simulink model "BUP_FOR_GUI"  (R2018a)
settings: Solver=ode3  StartTime=0.0  StopTime=1000  FixedStep=1  MinStep=1e-8  RelTol=1e-8
undefined symbols (not defined in the file or in its folder): DiscIntNeverNeededParam
libraries: BupSimulinkLibraries x22, simulink_extras x11, SignalEditorBlockLib x2
(part 1 of 2)
settings Model: EnablePacing=on  PacingRate=10  Creator=Юзер33  LastModifiedBy=User33
settings DataIOCC: SaveFormat=Array  OutputSaveName=P_lon
settings OptimizationCC: DefaultParameterBehavior=Inlined  UseDivisionForNetSlopeComputation=on  UseFloatMulNetSlope=on  InlineInvariantSignals=on  PassReuseOutputArgsAs=Individual arguments  ZeroExternalMemoryAtStartup=off  ZeroInternalMemoryAtStartup=off  NoFixptDivByZeroProtection=on  EfficientFloat2IntCast=on  LifeSpan=1  OptimizationLevel=level1  OptimizationCustomize=off
settings DebuggingCC: ParameterTunabilityLossMsg=error
settings HardwareCC: ProdBitPerPointer=32  ProdBitPerSizeT=32  ProdBitPerPtrDiffT=32  ProdLargestAtomicInteger=Long  ProdLargestAtomicFloat=Double  ProdWordSize=32  ProdLongLongMode=on  ProdHWDeviceType=ARM Compatible->ARM Cortex
settings SFSimCC: MATLABDynamicMemAlloc=off
settings RTWCC: SystemTargetFile=ert.tlc  GenCodeOnly=on  PackageGeneratedCodeAndArtifacts=on  PackageName=BupModel  TemplateMakefile=ert_default_tmf  GenerateReport=on  RTWVerbose=off  BuildConfiguration=Faster Runs  IncludeHyperlinkInReport=on  LaunchReport=on  GenerateTraceInfo=on  GenerateTraceReport=on  GenerateTraceReportSl=on  GenerateTraceReportSf=on  GenerateTraceReportEml=on  GenerateWebview=on  GenerateCodeMetricsReport=on  GenerateCodeReplacementReport=on
settings CodeAppCC: ForceParamTrailComments=on  IgnoreCustomStorageClasses=off  OperatorAnnotations=on  SimulinkDataObjDesc=on  SFDataObjDesc=on  MATLABFcnDesc=on  CustomSymbolStrGlobalVar=Easy_reg_$N$M  CustomSymbolStrType=$N$M  CustomSymbolStrFcn=$N$M$F  CustomSymbolStrMacro=$N$M  InsertBlockDesc=on  StateflowObjectComments=on  MATLABSourceComments=on  ReqsInCode=on
settings ERTTargetCC: TargetLangStandard=C99 (ISO)  GenerateSampleERTMain=on  IncludeMdlTerminateFcn=off  CombineSignalStateStructs=on  SupportComplex=off  SupportNonInlinedSFcns=on  InlinedParameterPlacement=NonHierarchical  RootIOFormat=Structure reference  ERTCustomFileTemplate=example_file_process.tlc  ERTFilePackagingFormat=CompactWithDataFile

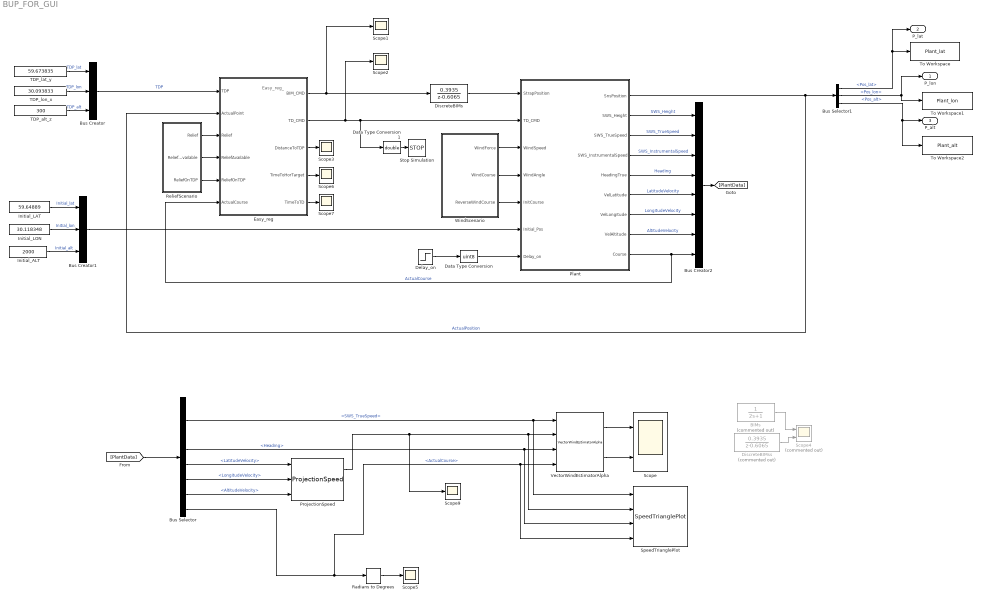
== system BUP_FOR_GUI ==
  note: Easy_reg_
  BIMs : TransferFcn  Commented=on  Denominator=[2 1]
  Bus Creator : BusCreator  Inputs=3
  Bus Creator1 : BusCreator  Inputs=3
  Bus Creator2 : BusCreator  Inputs=8
  Bus Selector : BusSelector  OutputSignals=SWS_Height,SWS_TrueSpeed,SWS_InstrumentalSpeed,Heading,LatitudeVelocity,LongitudeVelocity,AltitudeVelocity,ActualCourse
  Bus Selector1 : BusSelector  OutputSignals=Pos_lat,Pos_lon,Pos_alt
  Data Type Conversion : DataTypeConversion  OutDataTypeStr=uint8
  Data Type Conversion1 : DataTypeConversion  OutDataTypeStr=double
  Delay_on : Step  Time=20  SampleTime=0
  DiscreteBIMs : DiscreteTransferFcn  Numerator=[0.3935]  Denominator=[1 -0.6065]
  DiscreteBIMss : DiscreteTransferFcn  Commented=on  Numerator=[0.3935]  Denominator=[1 -0.6065]
  Easy_reg : Subsystem  TreatAsAtomicUnit=on  SystemSampleTime=1
  Initial_ALT : Constant  Value=2000
  Initial_LAT : Constant  Value=59.64889
  Initial_LON : Constant  Value=30.118348
  Plant : Subsystem  TreatAsAtomicUnit=on
  ProjectionSpeed : BupSimulinkLibraries/ProjectionSpeed
  Radians to Degrees : simulink_extras/Transformations/Radians to Degrees
  ReliefScenario : Subsystem  SystemSampleTime=1
  Scope : Scope  NumInputPorts=2
  Scope{1..3,5..7,9} (7 alike) : Scope
  Scope4 : Scope  Commented=on  NumInputPorts=2
  SpeedTrianglePlot : BupSimulinkLibraries/SpeedTrianglePlot
  Stop Simulation : Stop
  TDP_alt_z : Constant  Value=300
  TDP_lat_y : Constant  Value=59.673835
  TDP_lon_x : Constant  Value=30.093833
  To Workspace : ToWorkspace  VariableName=Plant_lat  SampleTime=-1
  To Workspace1 : ToWorkspace  VariableName=Plant_lon  SampleTime=-1
  To Workspace2 : ToWorkspace  VariableName=Plant_alt  SampleTime=-1
  VectorWindEstimatorAlpha : BupSimulinkLibraries/VectorWindEstimatorAlpha  SystemSampleTime=-1
  WindScenario : Subsystem  SystemSampleTime=1
  P_lon : Outport
  P_lat : Outport  Port=2
  P_alt : Outport  Port=3
  wires:
  TDP_alt_z/1 -> Bus Creator/3  "TDP_alt"
  TDP_lon_x/1 -> Bus Creator/2  "TDP_lon"
  TDP_lat_y/1 -> Bus Creator/1  "TDP_lat"
  Bus Creator/1 -> Easy_reg/1(TDP)  "TDP"
  Plant/1(SnsPosition) -> Easy_reg/2(ActualPoint), Bus Selector1/1  "ActualPosition"
  Initial_LAT/1 -> Bus Creator1/1  "Initial_lat"
  Bus Creator1/1 -> Plant/6(Initial_Pos)
  Initial_LON/1 -> Bus Creator1/2  "Initial_lon"
  Initial_ALT/1 -> Bus Creator1/3  "Initial_alt"
  BIMs/1 -> Scope4/1
  DiscreteBIMss/1 -> Scope4/2
  Bus Selector1/1 -> To Workspace/1, P_lat/1  "<Pos_lat>"
  Delay_on/1 -> Data Type Conversion/1
  ReliefScenario/3(ReliefOnTDP) -> Easy_reg/5(ReliefOnTDP)
  ReliefScenario/1(Relief) -> Easy_reg/3(Relief)
  ReliefScenario/2(ReliefAvailable) -> Easy_reg/4(ReliefAvailable)
  DiscreteBIMs/1 -> Plant/1(StrapPosition)
  Easy_reg/1(BIM_CMD) -> DiscreteBIMs/1, Scope1/1
  Easy_reg/2(TD_CMD) -> Scope2/1, Data Type Conversion1/1, Plant/2(TD_CMD)
  Data Type Conversion/1 -> Plant/7(Delay_on)
  Bus Selector1/2 -> P_lon/1, To Workspace1/1  "<Pos_lon>"
  Bus Selector1/3 -> To Workspace2/1, P_alt/1  "<Pos_alt>"
  Plant/7(VelLongitude) -> Bus Creator2/6  "LongitudeVelocity"
  Plant/8(VelAltitude) -> Bus Creator2/7  "AltitudeVelocity"
  Plant/6(VelLatitude) -> Bus Creator2/5  "LatitudeVelocity"
  Plant/2(SWS_Height) -> Bus Creator2/1  "SWS_Height"
  Plant/5(HeadingTrue) -> Bus Creator2/4  "Heading"
  Plant/4(SWS_InstrumentalSpeed) -> Bus Creator2/3  "SWS_InstrumentalSpeed"
  Bus Creator2/1 -> [PlantData]
  Plant/9(Course) -> Easy_reg/6(ActualCourse), Bus Creator2/8  "ActualCourse"
  Plant/3(SWS_TrueSpeed) -> Bus Creator2/2  "SWS_TrueSpeed"
  WindScenario/2(WindCourse) -> Plant/4(WindAngle)
  WindScenario/1(WindForce) -> Plant/3(WindSpeed)
  WindScenario/3(ReverseWindCourse) -> Plant/5(InitCourse)
  [PlantData] -> Bus Selector/1
  Bus Selector/6 -> ProjectionSpeed/2  "<LongitudeVelocity>"
  Bus Selector/2 -> SpeedTrianglePlot/1, VectorWindEstimatorAlpha/1  "<SWS_TrueSpeed>"
  Radians to Degrees/1 -> Scope5/1
  Bus Selector/8 -> SpeedTrianglePlot/4, VectorWindEstimatorAlpha/4, Radians to Degrees/1  "<ActualCourse>"
  Bus Selector/4 -> SpeedTrianglePlot/3, VectorWindEstimatorAlpha/3  "<Heading>"
  VectorWindEstimatorAlpha/1 -> Scope/1
  VectorWindEstimatorAlpha/2 -> Scope/2
  ProjectionSpeed/1 -> Scope9/1, SpeedTrianglePlot/2, VectorWindEstimatorAlpha/2
  Bus Selector/5 -> ProjectionSpeed/1  "<LatitudeVelocity>"
  Bus Selector/7 -> ProjectionSpeed/3  "<AltitudeVelocity>"
  Data Type Conversion1/1 -> Stop Simulation/1
  Easy_reg/3(DistanceToTDP) -> Scope3/1
  Easy_reg/4(TimeToHorTarget) -> Scope6/1
  Easy_reg/5(TimeToTD) -> Scope7/1

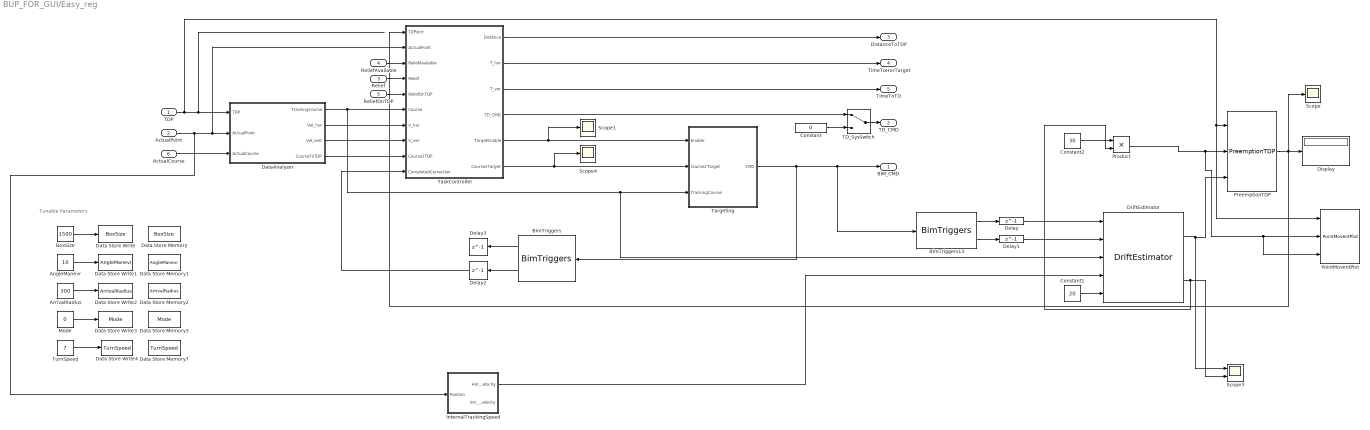
== system BUP_FOR_GUI/Easy_reg ==
  note: Tunable Parameters
  TDP : Inport
  ActualPoint : Inport  Port=2
  Relief : Inport  Port=3
  ReliefAvailable : Inport  Port=4
  ReliefOnTDP : Inport  Port=5
  ActualCourse : Inport  Port=6
  AngleManevr : Constant  Value=10
  ArrivalRadius : Constant  Value=300
  BimTriggers : BupSimulinkLibraries/BimTriggers
  BimTriggers13 : BupSimulinkLibraries/BimTriggers
  BoxSize : Constant  Value=1500
  Constant : Constant  Value=0
  Constant1 : Constant  Value=20
  Constant2 : Constant  Value=30
  Data Store Memory : DataStoreMemory  DataStoreName=BoxSize  ReadBeforeWriteMsg=warning  WriteAfterWriteMsg=warning  WriteAfterReadMsg=warning  ShowAdditionalParam=off  OutDataTypeStr=double  Dimensions=1
  Data Store Memory1 : DataStoreMemory  DataStoreName=AngleManevr  ReadBeforeWriteMsg=warning  WriteAfterWriteMsg=warning  WriteAfterReadMsg=warning  ShowAdditionalParam=off  OutDataTypeStr=double  Dimensions=1
  Data Store Memory2 : DataStoreMemory  DataStoreName=ArrivalRadius  ReadBeforeWriteMsg=warning  WriteAfterWriteMsg=warning  WriteAfterReadMsg=warning  ShowAdditionalParam=off  OutDataTypeStr=double  Dimensions=1
  Data Store Memory3 : DataStoreMemory  DataStoreName=Mode  ReadBeforeWriteMsg=warning  WriteAfterWriteMsg=warning  WriteAfterReadMsg=warning  ShowAdditionalParam=off  OutDataTypeStr=uint8  Dimensions=1
  Data Store Memory7 : DataStoreMemory  DataStoreName=TurnSpeed  ReadBeforeWriteMsg=warning  WriteAfterWriteMsg=warning  WriteAfterReadMsg=warning  ShowAdditionalParam=off  OutDataTypeStr=double  Dimensions=1
  Data Store Write : DataStoreWrite  DataStoreName=BoxSize
  Data Store Write1 : DataStoreWrite  DataStoreName=AngleManevr
  Data Store Write2 : DataStoreWrite  DataStoreName=ArrivalRadius
  Data Store Write3 : DataStoreWrite  DataStoreName=Mode
  Data Store Write4 : DataStoreWrite  DataStoreName=TurnSpeed
  DataAnalyzer : Subsystem
  Delay : Delay  DelayLength=1
  Delay1 : Delay  DelayLength=1
  Delay2 : Delay  DelayLength=1  InitialCondition=0
  Delay3 : Delay  DelayLength=1  InitialCondition=0
  Display : Display
  DriftEstimator : BupSimulinkLibraries/DriftEstimator
  InternalTrackingSpeed : Subsystem
  Mode : Constant  Value=0  OutDataTypeStr=uint8
  PointMoventPlot : BupSimulinkLibraries/PointMoventPlot
  PreemptionTDP : BupSimulinkLibraries/PreemptionTDP
  Product : Product
  Scope : Scope
  Scope1 : Scope
  Scope3 : Scope  NumInputPorts=2
  Scope4 : Scope
  TD_SysSwitch : ManualSwitch
  Targeting : Subsystem
  TaskController : Stateflow chart  TreatAsAtomicUnit=on  SystemSampleTime=1
  TurnSpeed : Constant  Value=7  OutDataTypeStr=double
  BIM_CMD : Outport
  TD_CMD : Outport  Port=2  OutDataTypeStr=uint8
  DistanceToTDP : Outport  Port=3
  TimeToHorTarget : Outport  Port=4
  TimeToTD : Outport  Port=5
  wires:
  TaskController/4(TD_CMD) -> TD_SysSwitch/1
  BoxSize/1 -> Data Store Write/1
  AngleManevr/1 -> Data Store Write1/1
  ArrivalRadius/1 -> Data Store Write2/1
  TD_SysSwitch/1 -> TD_CMD/1
  Constant/1 -> TD_SysSwitch/2
  Mode/1 -> Data Store Write3/1
  TurnSpeed/1 -> Data Store Write4/1
  TaskController/5(TargetEnable) -> Scope1/1, Targeting/1(Enable)
  DataAnalyzer/2(Vel_hor) -> TaskController/7(V_hor)
  DataAnalyzer/3(Vel_vert) -> TaskController/8(V_ver)
  ActualCourse/1 -> DataAnalyzer/3(ActualCourse)
  ReliefAvailable/1 -> TaskController/3(ReliefAvailable)
  Relief/1 -> TaskController/4(Relief)
  ReliefOnTDP/1 -> TaskController/5(ReliefOnTDP)
  TaskController/1(Distance) -> DistanceToTDP/1
  TaskController/2(T_hor) -> TimeToHorTarget/1
  TaskController/3(T_ver) -> TimeToTD/1
  ActualPoint/1 -> InternalTrackingSpeed/1(Position), DataAnalyzer/2(ActualPoint), TaskController/2(ActualPoint)
  TaskController/6(Course2Target) -> Scope4/1, Targeting/2(Course2Target)
  Targeting/1(CMD) -> BimTriggers/1, BimTriggers13/1, BIM_CMD/1
  Delay/1 -> DriftEstimator/1
  Delay1/1 -> DriftEstimator/2
  DriftEstimator/2 -> Product/2, Scope3/2
  BimTriggers13/2 -> Delay1/1
  BimTriggers13/1 -> Delay/1
  BimTriggers/2 -> Delay2/1
  TDP/1 -> PointMoventPlot/1, PreemptionTDP/1, DataAnalyzer/1(TDP)
  DataAnalyzer/1(TrackingCourse) -> DriftEstimator/3, Targeting/3(TrackingCourse), TaskController/6(Course)
  InternalTrackingSpeed/1(Hor_Velocity) -> DriftEstimator/4
  DataAnalyzer/4(CourseToTDP) -> TaskController/9(Course2TDP)
  DriftEstimator/1 -> PreemptionTDP/3, Scope3/1
  Constant1/1 -> DriftEstimator/5
  BimTriggers/1 -> Delay3/1
  Delay2/1 -> TaskController/10(CompletedCorrection)
  Constant2/1 -> Product/1
  Product/1 -> PointMoventPlot/3, PointMoventPlot/2, PreemptionTDP/2
  PreemptionTDP/1 -> Scope/1, TaskController/1(TDPoint), Display/1

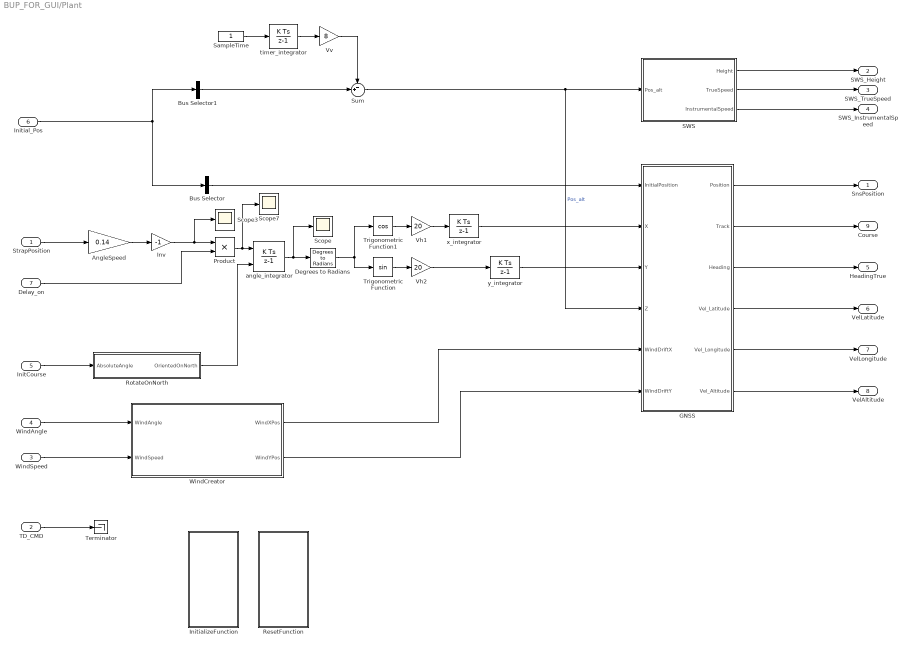
== system BUP_FOR_GUI/Plant ==
  StrapPosition : Inport  OutDataTypeStr=double  PortDimensions=1
  TD_CMD : Inport  Port=2  OutDataTypeStr=uint8  PortDimensions=1
  WindSpeed : Inport  Port=3
  WindAngle : Inport  Port=4
  InitCourse : Inport  Port=5
  Initial_Pos : Inport  Port=6
  Delay_on : Inport  Port=7
  AngleSpeed : Gain  Gain=0.14
  Bus Selector : BusSelector  OutputSignals=Initial_lat,Initial_lon  OutputAsBus=on
  Bus Selector1 : BusSelector  OutputSignals=Initial_alt  OutputAsBus=on
  Degrees to Radians : simulink_extras/Transformations/Degrees to Radians
  GNSS : Subsystem
  InitializeFunction : Subsystem  TreatAsAtomicUnit=on
  Inv : Gain  Gain=-1
  Product : Product
  ResetFunction : Subsystem  TreatAsAtomicUnit=on
  RotateOnNorth : Subsystem
  SWS : Subsystem
  SampleTime : Constant
  Scope : Scope
  Scope3 : Scope
  Scope7 : Scope
  Sum : Sum  Inputs=-+|
  Terminator : Terminator
  Trigonometric Function : Trigonometry
  Trigonometric Function1 : Trigonometry  Operator=cos
  Vh1 : Gain  Gain=20
  Vh2 : Gain  Gain=20
  Vv : Gain  Gain=8
  WindCreator : Subsystem
  angle_integrator : DiscreteIntegrator  InitialConditionSource=external  InitialCondition=90  SampleTime=-1  ICPrevOutput=DiscIntNeverNeededParam  ICPrevScaledInput=DiscIntNeverNeededParam
  timer_integrator : DiscreteIntegrator  SampleTime=-1  ICPrevOutput=DiscIntNeverNeededParam  ICPrevScaledInput=DiscIntNeverNeededParam
  x_integrator : DiscreteIntegrator  SampleTime=-1  ICPrevOutput=DiscIntNeverNeededParam  ICPrevScaledInput=DiscIntNeverNeededParam
  y_integrator : DiscreteIntegrator  SampleTime=-1  ICPrevOutput=DiscIntNeverNeededParam  ICPrevScaledInput=DiscIntNeverNeededParam
  SnsPosition : Outport
  SWS_Height : Outport  Port=2
  SWS_TrueSpeed : Outport  Port=3
  SWS_InstrumentalSpeed : Outport  Port=4
  HeadingTrue : Outport  Port=5
  VelLatitude : Outport  Port=6
  VelLongitude : Outport  Port=7
  VelAltitude : Outport  Port=8
  Course : Outport  Port=9
  wires:
  Degrees to Radians/1 -> Trigonometric Function1/1, Trigonometric Function/1
  angle_integrator/1 -> Scope/1, Degrees to Radians/1
  Trigonometric Function1/1 -> Vh1/1
  Trigonometric Function/1 -> Vh2/1
  Inv/1 -> Product/1, Scope3/1
  Delay_on/1 -> Product/2
  timer_integrator/1 -> Vv/1
  Vv/1 -> Sum/1
  Sum/1 -> GNSS/4(Z), SWS/1(Pos_alt)  "Pos_alt"
  Initial_Pos/1 -> Bus Selector1/1, Bus Selector/1
  Bus Selector/1 -> GNSS/1(InitialPosition)
  Bus Selector1/1 -> Sum/2
  Vh1/1 -> x_integrator/1
  Vh2/1 -> y_integrator/1
  StrapPosition/1 -> AngleSpeed/1
  Product/1 -> Scope7/1, angle_integrator/1
  AngleSpeed/1 -> Inv/1
  SWS/1(Height) -> SWS_Height/1
  SWS/2(TrueSpeed) -> SWS_TrueSpeed/1
  SWS/3(InstrumentalSpeed) -> SWS_InstrumentalSpeed/1
  SampleTime/1 -> timer_integrator/1
  InitCourse/1 -> RotateOnNorth/1(AbsoluteAngle)
  TD_CMD/1 -> Terminator/1
  WindAngle/1 -> WindCreator/1(WindAngle)
  WindSpeed/1 -> WindCreator/2(WindSpeed)
  RotateOnNorth/1(OrientedOnNorth) -> angle_integrator/2
  x_integrator/1 -> GNSS/2(X)
  y_integrator/1 -> GNSS/3(Y)
  WindCreator/1(WindXPos) -> GNSS/5(WindDriftX)
  WindCreator/2(WindYPos) -> GNSS/6(WindDriftY)
  GNSS/1(Position) -> SnsPosition/1
  GNSS/3(Heading) -> HeadingTrue/1
  GNSS/2(Track) -> Course/1
  GNSS/4(Vel_Latitude) -> VelLatitude/1
  GNSS/5(Vel_Longitude) -> VelLongitude/1
  GNSS/6(Vel_Altitude) -> VelAltitude/1

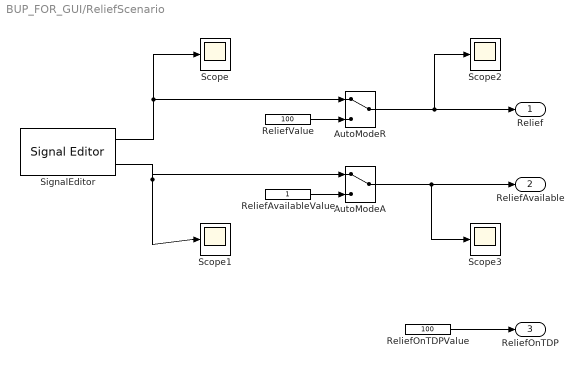
== system BUP_FOR_GUI/ReliefScenario ==
  AutoModeA : ManualSwitch
  AutoModeR : ManualSwitch
  ReliefAvailableValue : Constant  OutDataTypeStr=uint8
  ReliefOnTDPValue : Constant  Value=100  OutDataTypeStr=int16
  ReliefValue : Constant  Value=100  OutDataTypeStr=int16
  Scope{,1..3} (4 alike) : Scope
  SignalEditor : SignalEditorBlockLib/Signal Editor  FileName=ReliefScenario.mat  ActiveScenario=Scenario  ActiveSignal=Relief  IsBus=off  OutputBusObjectStr=Bus: BusObject  SampleTime=-1  ZeroCross=off  OutputAfterFinalValue=Setting to zero  Unit=inherit
  Relief : Outport
  ReliefAvailable : Outport  Port=2
  ReliefOnTDP : Outport  Port=3
  wires:
  SignalEditor/2 -> Scope1/1, AutoModeA/1
  SignalEditor/1 -> Scope/1, AutoModeR/1
  ReliefAvailableValue/1 -> AutoModeA/2
  ReliefValue/1 -> AutoModeR/2
  AutoModeR/1 -> Scope2/1, Relief/1
  AutoModeA/1 -> Scope3/1, ReliefAvailable/1
  ReliefOnTDPValue/1 -> ReliefOnTDP/1

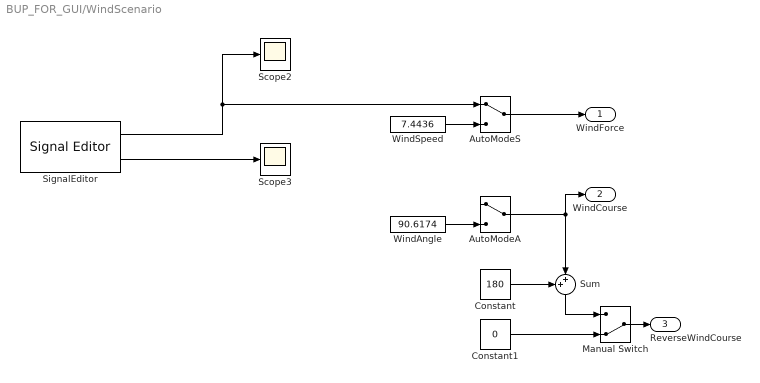
== system BUP_FOR_GUI/WindScenario ==
  AutoModeA : ManualSwitch
  AutoModeS : ManualSwitch
  Constant : Constant  Value=180
  Constant1 : Constant  Value=0
  Manual Switch : ManualSwitch  CurrentSetting=0
  Scope2 : Scope
  Scope3 : Scope
  SignalEditor : SignalEditorBlockLib/Signal Editor  FileName=autoWind.mat  ActiveScenario=Scenario  ActiveSignal=WindSpeed  IsBus=off  OutputBusObjectStr=Bus: BusObject  SampleTime=-1  ZeroCross=off  OutputAfterFinalValue=Setting to zero  Unit=inherit
  Sum : Sum  Inputs=++|
  WindAngle : Constant  Value=90.6174
  WindSpeed : Constant  Value=7.4436
  WindForce : Outport
  WindCourse : Outport  Port=2
  ReverseWindCourse : Outport  Port=3
  wires:
  SignalEditor/1 -> AutoModeS/1, Scope2/1
  WindAngle/1 -> AutoModeA/2
  WindSpeed/1 -> AutoModeS/2
  AutoModeS/1 -> WindForce/1
  AutoModeA/1 -> WindCourse/1, Sum/2
  Sum/1 -> Manual Switch/1
  Constant/1 -> Sum/1
  Manual Switch/1 -> ReverseWindCourse/1
  Constant1/1 -> Manual Switch/2
  SignalEditor/2 -> Scope3/1

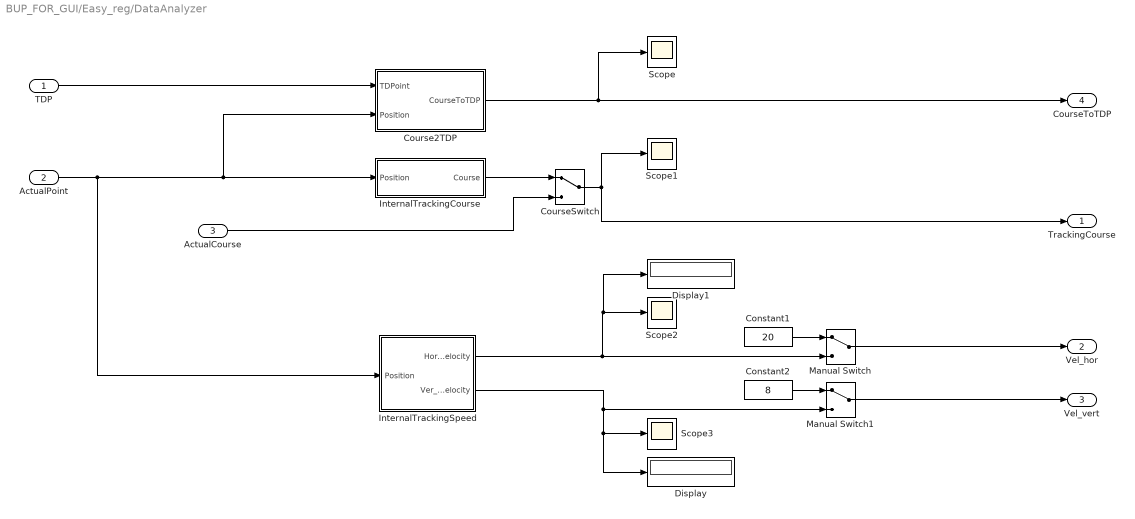
== system BUP_FOR_GUI/Easy_reg/DataAnalyzer ==
  TDP : Inport
  ActualPoint : Inport  Port=2
  ActualCourse : Inport  Port=3
  Constant1 : Constant  Value=20
  Constant2 : Constant  Value=8
  Course2TDP : Subsystem
  CourseSwitch : ManualSwitch
  Display : Display
  Display1 : Display
  InternalTrackingCourse : Subsystem
  InternalTrackingSpeed : Subsystem
  Manual Switch : ManualSwitch
  Manual Switch1 : ManualSwitch
  Scope{,1..3} (4 alike) : Scope
  TrackingCourse : Outport
  Vel_hor : Outport  Port=2
  Vel_vert : Outport  Port=3
  CourseToTDP : Outport  Port=4
  wires:
  CourseSwitch/1 -> TrackingCourse/1, Scope1/1
  TDP/1 -> Course2TDP/1(TDPoint)
  InternalTrackingCourse/1(Course) -> CourseSwitch/1
  ActualCourse/1 -> CourseSwitch/2
  ActualPoint/1 -> InternalTrackingSpeed/1(Position), Course2TDP/2(Position), InternalTrackingCourse/1(Position)
  InternalTrackingSpeed/1(Hor_Velocity) -> Manual Switch/2, Display1/1, Scope2/1
  InternalTrackingSpeed/2(Ver_Velocity) -> Manual Switch1/2, Scope3/1, Display/1
  Manual Switch/1 -> Vel_hor/1
  Constant1/1 -> Manual Switch/1
  Manual Switch1/1 -> Vel_vert/1
  Course2TDP/1(CourseToTDP) -> Scope/1, CourseToTDP/1
  Constant2/1 -> Manual Switch1/1

== system BUP_FOR_GUI/Easy_reg/InternalTrackingSpeed ==
  Position : Inport
  Constant : Constant
  GPSVelocity : BupSimulinkLibraries/GPSVelocity
  LastPos1 : Delay  DelayLength=1
  ProjectionSpeed : BupSimulinkLibraries/ProjectionSpeed
  Hor_Velocity : Outport
  Ver_Velocity : Outport  Port=2
  wires:
  LastPos1/1 -> GPSVelocity/2
  ProjectionSpeed/2 -> Ver_Velocity/1
  Position/1 -> LastPos1/1, GPSVelocity/1
  ProjectionSpeed/1 -> Hor_Velocity/1
  GPSVelocity/1 -> ProjectionSpeed/1
  GPSVelocity/2 -> ProjectionSpeed/2
  GPSVelocity/3 -> ProjectionSpeed/3
  Constant/1 -> GPSVelocity/3

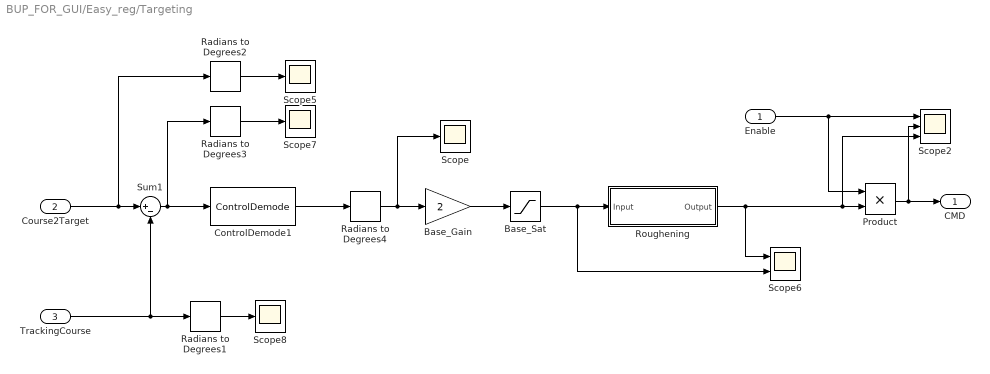
== system BUP_FOR_GUI/Easy_reg/Targeting ==
  Enable : Inport  OutDataTypeStr=uint8  PortDimensions=1
  Course2Target : Inport  Port=2  OutDataTypeStr=double  PortDimensions=1
  TrackingCourse : Inport  Port=3  OutDataTypeStr=double  PortDimensions=1
  Base_Gain : Gain  Gain=2
  Base_Sat : Saturate  UpperLimit=50  LowerLimit=-50
  ControlDemode1 : BupSimulinkLibraries/ControlDemode
  Product : Product
  Radians to Degrees{1..4} (4 alike) : simulink_extras/Transformations/Radians to Degrees
  Roughening : Subsystem
  Scope{,5,7..8} (4 alike) : Scope
  Scope2 : Scope  NumInputPorts=3
  Scope6 : Scope  NumInputPorts=2
  Sum1 : Sum  Inputs=|+-
  CMD : Outport  OutDataTypeStr=double
  wires:
  Course2Target/1 -> Radians to Degrees2/1, Sum1/1
  Radians to Degrees3/1 -> Scope7/1
  Radians to Degrees2/1 -> Scope5/1
  Base_Sat/1 -> Scope6/2, Roughening/1(Input)
  Base_Gain/1 -> Base_Sat/1
  Radians to Degrees4/1 -> Scope/1, Base_Gain/1
  Enable/1 -> Product/1, Scope2/1
  Product/1 -> Scope2/2, CMD/1
  TrackingCourse/1 -> Radians to Degrees1/1, Sum1/2
  Sum1/1 -> ControlDemode1/1, Radians to Degrees3/1
  ControlDemode1/1 -> Radians to Degrees4/1
  Roughening/1(Output) -> Product/2, Scope2/3, Scope6/1
  Radians to Degrees1/1 -> Scope8/1

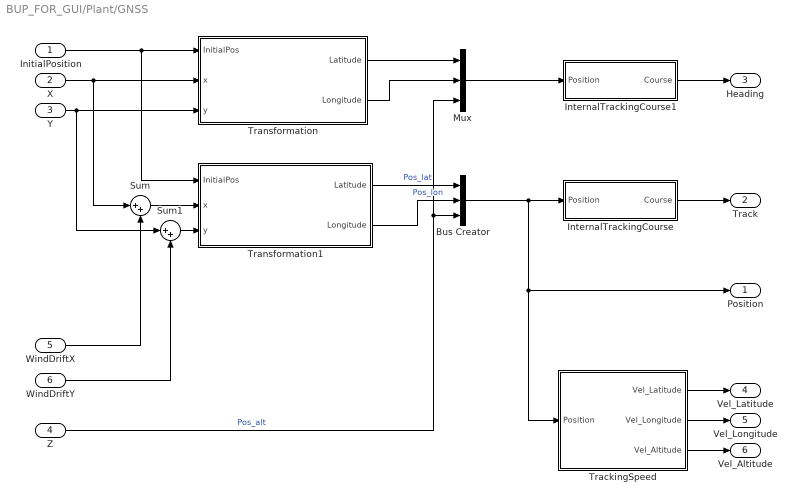
== system BUP_FOR_GUI/Plant/GNSS ==
  InitialPosition : Inport
  X : Inport  Port=2
  Y : Inport  Port=3
  Z : Inport  Port=4
  WindDriftX : Inport  Port=5
  WindDriftY : Inport  Port=6
  Bus Creator : BusCreator  Inputs=3
  InternalTrackingCourse : Subsystem
  InternalTrackingCourse1 : Subsystem
  Mux : Mux  Inputs=3
  Sum : Sum  Inputs=|++
  Sum1 : Sum  Inputs=|++
  TrackingSpeed : Subsystem
  Transformation : Subsystem
  Transformation1 : Subsystem
  Position : Outport
  Track : Outport  Port=2
  Heading : Outport  Port=3
  Vel_Latitude : Outport  Port=4
  Vel_Longitude : Outport  Port=5
  Vel_Altitude : Outport  Port=6
  wires:
  InitialPosition/1 -> Transformation1/1(InitialPos), Transformation/1(InitialPos)
  X/1 -> Sum/1, Transformation/2(x)
  Y/1 -> Sum1/1, Transformation/3(y)
  Sum/1 -> Transformation1/2(x)
  Sum1/1 -> Transformation1/3(y)
  WindDriftX/1 -> Sum/2
  WindDriftY/1 -> Sum1/2
  TrackingSpeed/2(Vel_Longitude) -> Vel_Longitude/1
  TrackingSpeed/3(Vel_Altitude) -> Vel_Altitude/1
  TrackingSpeed/1(Vel_Latitude) -> Vel_Latitude/1
  Transformation/1(Latitude) -> Mux/1
  Transformation/2(Longitude) -> Mux/2
  Mux/1 -> InternalTrackingCourse1/1(Position)
  Transformation1/1(Latitude) -> Bus Creator/1  "Pos_lat"
  Bus Creator/1 -> InternalTrackingCourse/1(Position), TrackingSpeed/1(Position), Position/1
  Z/1 -> Mux/3, Bus Creator/3  "Pos_alt"
  InternalTrackingCourse1/1(Course) -> Heading/1
  InternalTrackingCourse/1(Course) -> Track/1
  Transformation1/2(Longitude) -> Bus Creator/2  "Pos_lon"

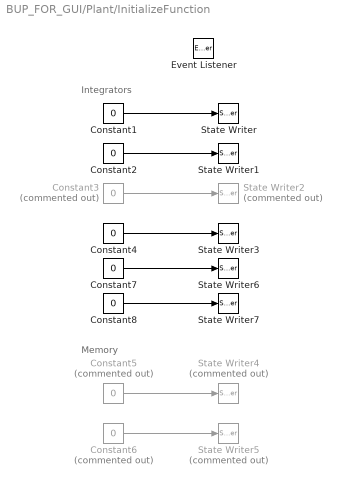
== system BUP_FOR_GUI/Plant/InitializeFunction ==
  note: Memory
  note: Integrators
  Constant{1..2,4,7..8} (5 alike) : Constant  Value=0
  Constant3 : Constant  Commented=on  Value=0
  Constant5 : Constant  Commented=on  Value=0
  Constant6 : Constant  Commented=on  Value=0
  Event Listener : EventListener  DisableCoverage=on  EventName=reset
  State Writer : StateWriter  StateOwnerBlock=../../x_integrator
  State Writer1 : StateWriter  StateOwnerBlock=../../y_integrator
  State Writer2 : StateWriter  Commented=on  StateOwnerBlock=../../angle_integrator
  State Writer3 : StateWriter  StateOwnerBlock=../../timer_integrator
  State Writer4 : StateWriter  Commented=on
  State Writer5 : StateWriter  Commented=on
  State Writer6 : StateWriter  StateOwnerBlock=../../WindCreator/WindXintegrator
  State Writer7 : StateWriter  StateOwnerBlock=../../WindCreator/WindYintegrator
  wires:
  Constant1/1 -> State Writer/1
  Constant2/1 -> State Writer1/1
  Constant3/1 -> State Writer2/1
  Constant4/1 -> State Writer3/1
  Constant5/1 -> State Writer4/1
  Constant6/1 -> State Writer5/1
  Constant7/1 -> State Writer6/1
  Constant8/1 -> State Writer7/1

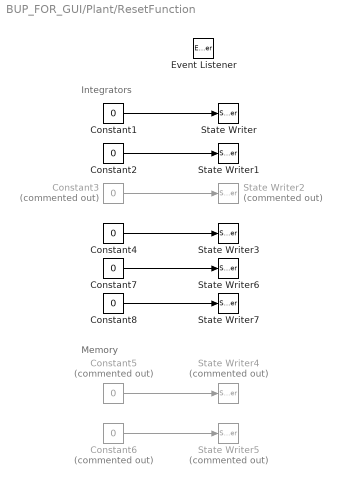
== system BUP_FOR_GUI/Plant/ResetFunction ==
  note: Memory
  note: Integrators
  Constant{1..2,4,7..8} (5 alike) : Constant  Value=0
  Constant3 : Constant  Commented=on  Value=0
  Constant5 : Constant  Commented=on  Value=0
  Constant6 : Constant  Commented=on  Value=0
  Event Listener : EventListener  DisableCoverage=on  EventType=Reset  EventName=reset
  State Writer : StateWriter  StateOwnerBlock=../../x_integrator
  State Writer1 : StateWriter  StateOwnerBlock=../../y_integrator
  State Writer2 : StateWriter  Commented=on  StateOwnerBlock=../../angle_integrator
  State Writer3 : StateWriter  StateOwnerBlock=../../timer_integrator
  State Writer4 : StateWriter  Commented=on
  State Writer5 : StateWriter  Commented=on
  State Writer6 : StateWriter  StateOwnerBlock=../../WindCreator/WindXintegrator
  State Writer7 : StateWriter  StateOwnerBlock=../../WindCreator/WindYintegrator
  wires:
  Constant1/1 -> State Writer/1
  Constant2/1 -> State Writer1/1
  Constant3/1 -> State Writer2/1
  Constant4/1 -> State Writer3/1
  Constant5/1 -> State Writer4/1
  Constant6/1 -> State Writer5/1
  Constant7/1 -> State Writer6/1
  Constant8/1 -> State Writer7/1

== system BUP_FOR_GUI/Plant/RotateOnNorth ==
  AbsoluteAngle : Inport
  Constant : Constant  Value=90
  Gain : Gain  Gain=-1
  Sum3 : Sum  Inputs=|+-
  OrientedOnNorth : Outport
  wires:
  AbsoluteAngle/1 -> Sum3/1
  Constant/1 -> Sum3/2
  Sum3/1 -> Gain/1
  Gain/1 -> OrientedOnNorth/1

== system BUP_FOR_GUI/Plant/SWS ==
  Pos_alt : Inport
  Constant : Constant  Value=20
  Constant1 : Constant  Value=20
  Constant2 : Constant  Value=20
  Sum3 : Sum  Inputs=++|
  Height : Outport
  TrueSpeed : Outport  Port=2
  InstrumentalSpeed : Outport  Port=3
  wires:
  Sum3/1 -> Height/1
  Constant/1 -> Sum3/1
  Pos_alt/1 -> Sum3/2
  Constant1/1 -> TrueSpeed/1
  Constant2/1 -> InstrumentalSpeed/1

== system BUP_FOR_GUI/Plant/WindCreator ==
  WindAngle : Inport
  WindSpeed : Inport  Port=2
  Degrees to Radians1 : simulink_extras/Transformations/Degrees to Radians
  Product1 : Product
  Product2 : Product
  RotateOnNorth : Subsystem
  Trigonometric Function2 : Trigonometry  Operator=cos
  Trigonometric Function3 : Trigonometry
  WindXintegrator : DiscreteIntegrator  SampleTime=-1  ICPrevOutput=DiscIntNeverNeededParam  ICPrevScaledInput=DiscIntNeverNeededParam
  WindYintegrator : DiscreteIntegrator  SampleTime=-1  ICPrevOutput=DiscIntNeverNeededParam  ICPrevScaledInput=DiscIntNeverNeededParam
  WindXPos : Outport
  WindYPos : Outport  Port=2
  wires:
  Product1/1 -> WindYintegrator/1
  WindSpeed/1 -> Product1/2, Product2/2
  Trigonometric Function2/1 -> Product2/1
  RotateOnNorth/1(OrientedOnNorth) -> Degrees to Radians1/1
  Trigonometric Function3/1 -> Product1/1
  Degrees to Radians1/1 -> Trigonometric Function3/1, Trigonometric Function2/1
  WindAngle/1 -> RotateOnNorth/1(AbsoluteAngle)
  Product2/1 -> WindXintegrator/1
  WindYintegrator/1 -> WindYPos/1
  WindXintegrator/1 -> WindXPos/1

== system BUP_FOR_GUI/Easy_reg/DataAnalyzer/Course2TDP ==
  TDPoint : Inport
  Position : Inport  Port=2
  Bearing : BupSimulinkLibraries/Bearing
  CourseToTDP : Outport
  wires:
  Position/1 -> Bearing/2
  TDPoint/1 -> Bearing/1
  Bearing/1 -> CourseToTDP/1

== system BUP_FOR_GUI/Easy_reg/DataAnalyzer/InternalTrackingCourse ==
  Position : Inport  OutDataTypeStr=double  PortDimensions=3
  Azimuth : BupSimulinkLibraries/Azimuth
  Bearing : BupSimulinkLibraries/Bearing
  Display : Display
  Display1 : Display
  LastPos : Delay  DelayLength=1
  Manual Switch2 : ManualSwitch
  Radians to Degrees1 : simulink_extras/Transformations/Radians to Degrees
  Radians to Degrees2 : simulink_extras/Transformations/Radians to Degrees
  Scope1 : Scope  NumInputPorts=2
  Scope8 : Scope
  Scope9 : Scope
  Course : Outport  OutDataTypeStr=double  PortDimensions=1
  wires:
  Bearing/1 -> Manual Switch2/1, Display/1, Radians to Degrees1/1, Scope8/1
  Azimuth/1 -> Manual Switch2/2, Scope9/1, Radians to Degrees2/1, Display1/1
  Manual Switch2/1 -> Course/1
  LastPos/1 -> Azimuth/2, Bearing/2
  Position/1 -> LastPos/1, Bearing/1, Azimuth/1
  Radians to Degrees1/1 -> Scope1/1
  Radians to Degrees2/1 -> Scope1/2

== system BUP_FOR_GUI/Easy_reg/DataAnalyzer/InternalTrackingSpeed ==
  Position : Inport
  Constant : Constant
  GPSVelocity : BupSimulinkLibraries/GPSVelocity
  LastPos1 : Delay  DelayLength=1
  ProjectionSpeed : BupSimulinkLibraries/ProjectionSpeed
  Hor_Velocity : Outport
  Ver_Velocity : Outport  Port=2
  wires:
  LastPos1/1 -> GPSVelocity/2
  ProjectionSpeed/2 -> Ver_Velocity/1
  Position/1 -> LastPos1/1, GPSVelocity/1
  ProjectionSpeed/1 -> Hor_Velocity/1
  GPSVelocity/1 -> ProjectionSpeed/1
  GPSVelocity/2 -> ProjectionSpeed/2
  GPSVelocity/3 -> ProjectionSpeed/3
  Constant/1 -> GPSVelocity/3

== system BUP_FOR_GUI/Easy_reg/Targeting/Roughening ==
  Input : Inport
  DeadZone : BupSimulinkLibraries/DeadZone
  Gain : Gain  Gain=0.1
  Gain1 : Gain  Gain=10
  Manual Switch : ManualSwitch  CurrentSetting=0
  Rounding Function : Rounding
  Scope : Scope  NumInputPorts=3
  Output : Outport
  wires:
  Input/1 -> Manual Switch/2, Scope/3, Gain/1
  Gain/1 -> Rounding Function/1
  Rounding Function/1 -> Gain1/1
  Gain1/1 -> Scope/1, DeadZone/1
  DeadZone/1 -> Manual Switch/1, Scope/2
  Manual Switch/1 -> Output/1

== system BUP_FOR_GUI/Plant/GNSS/InternalTrackingCourse ==
  Position : Inport  OutDataTypeStr=double  PortDimensions=3
  Azimuth : BupSimulinkLibraries/Azimuth
  Bearing : BupSimulinkLibraries/Bearing
  Display : Display
  Display1 : Display
  LastPos : Memory  InheritSampleTime=on
  Manual Switch2 : ManualSwitch
  Scope1 : Scope  NumInputPorts=2
  Scope8 : Scope
  Scope9 : Scope
  Course : Outport  OutDataTypeStr=double  PortDimensions=1
  wires:
  Bearing/1 -> Scope1/1, Display/1, Manual Switch2/1, Scope8/1
  Azimuth/1 -> Display1/1, Scope1/2, Manual Switch2/2, Scope9/1
  Manual Switch2/1 -> Course/1
  LastPos/1 -> Azimuth/2, Bearing/2
  Position/1 -> LastPos/1, Bearing/1, Azimuth/1

== system BUP_FOR_GUI/Plant/GNSS/InternalTrackingCourse1 ==
  Position : Inport  OutDataTypeStr=double  PortDimensions=3
  Azimuth : BupSimulinkLibraries/Azimuth
  Bearing : BupSimulinkLibraries/Bearing
  Display : Display
  Display1 : Display
  LastPos : Memory  InheritSampleTime=on
  Manual Switch2 : ManualSwitch
  Scope1 : Scope  NumInputPorts=2
  Scope8 : Scope
  Scope9 : Scope
  Course : Outport  OutDataTypeStr=double  PortDimensions=1
  wires:
  Bearing/1 -> Scope1/1, Display/1, Manual Switch2/1, Scope8/1
  Azimuth/1 -> Display1/1, Scope1/2, Manual Switch2/2, Scope9/1
  Manual Switch2/1 -> Course/1
  LastPos/1 -> Azimuth/2, Bearing/2
  Position/1 -> LastPos/1, Bearing/1, Azimuth/1

== system BUP_FOR_GUI/Plant/GNSS/TrackingSpeed ==
  Position : Inport
  Constant : Constant
  GPSVelocity : BupSimulinkLibraries/GPSVelocity
  LastPos : Memory  InheritSampleTime=on  LinearizeAsDelay=on
  Vel_Latitude : Outport
  Vel_Longitude : Outport  Port=2
  Vel_Altitude : Outport  Port=3
  wires:
  LastPos/1 -> GPSVelocity/2
  Position/1 -> GPSVelocity/1, LastPos/1
  Constant/1 -> GPSVelocity/3
  GPSVelocity/3 -> Vel_Altitude/1
  GPSVelocity/2 -> Vel_Longitude/1
  GPSVelocity/1 -> Vel_Latitude/1

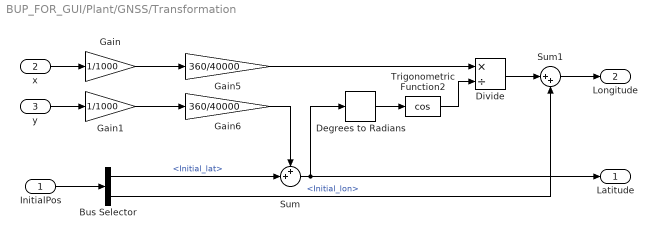
== system BUP_FOR_GUI/Plant/GNSS/Transformation ==
  InitialPos : Inport
  x : Inport  Port=2
  y : Inport  Port=3
  Bus Selector : BusSelector  OutputSignals=Initial_lat,Initial_lon
  Degrees to Radians : simulink_extras/Transformations/Degrees to Radians
  Divide : Product  Inputs=*/
  Gain : Gain  Gain=1/1000
  Gain1 : Gain  Gain=1/1000
  Gain5 : Gain  Gain=360/40000
  Gain6 : Gain  Gain=360/40000
  Sum : Sum  Inputs=++|
  Sum1 : Sum  Inputs=|++
  Trigonometric Function2 : Trigonometry  Operator=cos
  Latitude : Outport
  Longitude : Outport  Port=2
  wires:
  Divide/1 -> Sum1/1
  Gain5/1 -> Divide/1
  y/1 -> Gain1/1
  Gain6/1 -> Sum/1
  x/1 -> Gain/1
  Trigonometric Function2/1 -> Divide/2
  Degrees to Radians/1 -> Trigonometric Function2/1
  Gain/1 -> Gain5/1
  Gain1/1 -> Gain6/1
  InitialPos/1 -> Bus Selector/1
  Bus Selector/1 -> Sum/2  "<Initial_lat>"
  Bus Selector/2 -> Sum1/2  "<Initial_lon>"
  Sum/1 -> Degrees to Radians/1, Latitude/1
  Sum1/1 -> Longitude/1

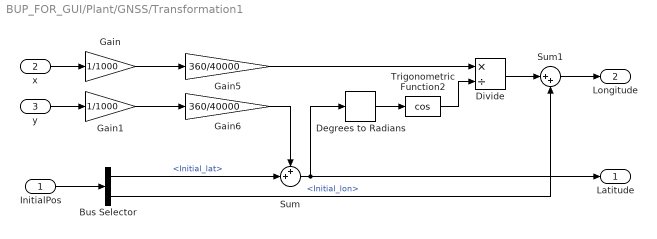
== system BUP_FOR_GUI/Plant/GNSS/Transformation1 ==
  InitialPos : Inport
  x : Inport  Port=2
  y : Inport  Port=3
  Bus Selector : BusSelector  OutputSignals=Initial_lat,Initial_lon
  Degrees to Radians : simulink_extras/Transformations/Degrees to Radians
  Divide : Product  Inputs=*/
  Gain : Gain  Gain=1/1000
  Gain1 : Gain  Gain=1/1000
  Gain5 : Gain  Gain=360/40000
  Gain6 : Gain  Gain=360/40000
  Sum : Sum  Inputs=++|
  Sum1 : Sum  Inputs=|++
  Trigonometric Function2 : Trigonometry  Operator=cos
  Latitude : Outport
  Longitude : Outport  Port=2
  wires:
  Sum1/1 -> Longitude/1
  Sum/1 -> Latitude/1, Degrees to Radians/1
  Bus Selector/2 -> Sum1/2  "<Initial_lon>"
  Bus Selector/1 -> Sum/2  "<Initial_lat>"
  InitialPos/1 -> Bus Selector/1
  Gain1/1 -> Gain6/1
  Gain/1 -> Gain5/1
  Degrees to Radians/1 -> Trigonometric Function2/1
  Trigonometric Function2/1 -> Divide/2
  x/1 -> Gain/1
  Gain6/1 -> Sum/1
  y/1 -> Gain1/1
  Gain5/1 -> Divide/1
  Divide/1 -> Sum1/1

== system BUP_FOR_GUI/Plant/WindCreator/RotateOnNorth ==
  AbsoluteAngle : Inport
  Constant : Constant  Value=90
  Gain : Gain  Gain=-1
  Sum3 : Sum  Inputs=|+-
  OrientedOnNorth : Outport
  wires:
  AbsoluteAngle/1 -> Sum3/1
  Constant/1 -> Sum3/2
  Sum3/1 -> Gain/1
  Gain/1 -> OrientedOnNorth/1
